simulink model "swing_up_final"  (R2020b)
settings: Solver=FixedStepDiscrete  StartTime=0.0  StopTime=Inf  FixedStep=0.001  RelTol=1e-3  EnableMultiTasking=on
values from neighbouring files (symbols this model uses):
  alfaBest = sin(2*pi*tacc/Tperiod)    [demo.m]    (also in pendulo_modelo.m)
  Gtd = c2d(Gt,T,'Tustin')    [demo.m]    (also in pendulo_modelo.m)
  Robs = [1 0 ... (first row only)    [demo.m]    (also in pendulo_modelo.m)
  Xmax = 0.02    [demo.m]    (also in pendulo_modelo.m = 0.045)
  Xmin = -0.02    [demo.m]    (also in pendulo_modelo.m = -0.045)
undefined symbols (not defined in the file or in its folder): DiscIntNeverNeededParam, Discrete, Kservo2, Time
libraries: simulink x5, arduinolib x2, ctrlSharedLib x1
settings Model: SILPILModeSetting=veronly  ExtModeTrigDuration=2  Creator=aleca  LastModifiedBy=aleca
settings OptimizationCC: EnhancedBackFolding=on  PassReuseOutputArgsAs=Individual arguments  ZeroExternalMemoryAtStartup=off  ZeroInternalMemoryAtStartup=off  MaxStackSize=64  OptimizeBlockOrder=speed  DifferentSizesBufferReuse=on  OptimizationCustomize=off  EfficientTunableParamExpr=on
settings DebuggingCC: ParameterTunabilityLossMsg=error
settings HardwareCC: ProdBitPerInt=16  ProdBitPerPointer=16  ProdBitPerSizeT=16  ProdBitPerPtrDiffT=16  ProdLargestAtomicFloat=None  ProdWordSize=8  ProdHWDeviceType=Atmel->AVR  UseEmbeddedCoderFeatures=off  UseSimulinkCoderFeatures=off
settings SFSimCC: MATLABDynamicMemAlloc=off
settings RTWCC: Description=Embedded Coder  SystemTargetFile=ert.tlc  HardwareBoard=Arduino Mega 2560  TemplateMakefile=ert_default_tmf  Toolchain=Arduino AVR  BuildConfiguration=Faster Runs
settings CodeAppCC: ForceParamTrailComments=on  IgnoreCustomStorageClasses=off  OperatorAnnotations=on  SimulinkDataObjDesc=on  SFDataObjDesc=on  InsertBlockDesc=on
settings ERTTargetCC: SupportContinuousTime=on  SupportNonInlinedSFcns=on  SupportVariableSizeSignals=on  ExtModeStaticAllocSize=2048

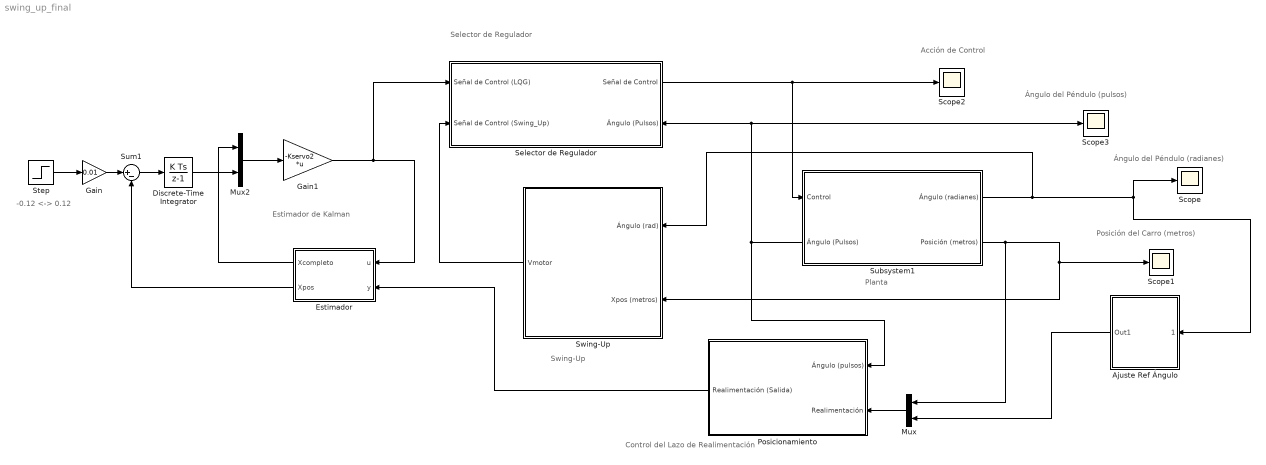
== system swing_up_final ==
  note: Selector de Regulador
  note: Posición del Carro (metros)
  note: Ángulo del Péndulo (radianes)
  note: Acción de Control
  note: Planta
  note: Ángulo del Péndulo (pulsos)
  note: Estimador de
      | Kalman
  note: Control del Lazo
      | de Realimentación
  note: -0.12 <-> 0.12
  note: Swing-Up
  Ajuste Ref Ángulo : Subsystem
  Discrete-Time Integrator : DiscreteIntegrator  SampleTime=-1  ICPrevOutput=DiscIntNeverNeededParam  ICPrevScaledInput=DiscIntNeverNeededParam
  Estimador : Subsystem
  Gain : Gain  Gain=0.01
  Gain1 : Gain  Gain=-Kservo2  Multiplication=Matrix(K*u)
  Mux : Mux  Inputs=2
  Mux2 : Mux  Inputs=2
  Posicionamiento : Subsystem
  Scope{,1..3} (4 alike) : Scope
  Selector de Regulador : Subsystem
      settings: PortSchema="{\"entries\":[{\"content\":{\"sides\":[{\"content\":{\"connectorIds\":[\"In1\",\"In2\"]},\"type\":\"ConnectorPlacement.EquallySpacedRectSide\",\"uuid\":\"3db4eb14-0c6e-4ec4-aee9-eaca3967a293\"},{\"content\":{\"connectorIds\":[\"Out1\",\"In3\"],\"side\":\"RIGHT\"},\"type\":\"ConnectorPlacement.EquallySpacedRectSide\",\"uuid\":\"3f8b5f83-bad3-4980-a559-890a6b6b79dc\"},{\"content\":{\"connectorIds\":[],\"side\":\"TOP\"},\"type\":\"ConnectorPlacement.EquallySpacedRectSide\",\"uuid\":\"0b873bda-4a27-449b-90e9-0421a7079439\"},{\"content\":{\"connectorIds\":[],\"side\":\"HIDDEN\"},\"type\":\"ConnectorPlacement.EquallySpacedRectSide\",\"uuid\":\"6335c064-abb3-4cb7-b774-07e736eb33ab\"}]},\"type\":\"ConnectorPlacement.EquallySpacedConnector\",\"uuid\":\"66807109-8b2f-4e1e-ad0b-5b86e298b8b1\"}],\"packageUris\":[\"http://schema.mathworks.com/mf0/Connector/R2020b\"],\"version\":\"1.0\"}"
  Step : Step  After=0  SampleTime=0.001
  Subsystem1 : Subsystem
      settings: PortSchema="{\"entries\":[{\"content\":{\"sides\":[{\"content\":{\"connectorIds\":[\"In1\",\"Out3\"]},\"type\":\"ConnectorPlacement.EquallySpacedRectSide\",\"uuid\":\"7b7d0a7e-b440-45e8-a961-32fe078fe659\"},{\"content\":{\"connectorIds\":[\"Out1\",\"Out2\"],\"side\":\"RIGHT\"},\"type\":\"ConnectorPlacement.EquallySpacedRectSide\",\"uuid\":\"86b71336-2b65-464f-a731-f6d3e5fd47fb\"},{\"content\":{\"connectorIds\":[],\"side\":\"TOP\"},\"type\":\"ConnectorPlacement.EquallySpacedRectSide\",\"uuid\":\"9d97f193-f97d-41ca-a241-68d679627dc2\"},{\"content\":{\"connectorIds\":[],\"side\":\"HIDDEN\"},\"type\":\"ConnectorPlacement.EquallySpacedRectSide\",\"uuid\":\"10f5410f-7265-49a9-9109-a49fd87294e3\"}]},\"type\":\"ConnectorPlacement.EquallySpacedConnector\",\"uuid\":\"71c4b2f0-2d03-4cb3-b067-cb634b3b5bca\"}],\"packageUris\":[\"http://schema.mathworks.com/mf0/Connector/R2020b\"],\"version\":\"1.0\"}"
  Sum1 : Sum  Inputs=|+-
  Swing-Up : Subsystem
      settings: PortSchema="{\"entries\":[{\"content\":{\"sides\":[{\"content\":{\"connectorIds\":[\"Out1\"]},\"type\":\"ConnectorPlacement.EquallySpacedRectSide\",\"uuid\":\"b2f1a7f6-c998-4070-93e8-aa818857c465\"},{\"content\":{\"connectorIds\":[\"In1\",\"In2\"],\"side\":\"RIGHT\"},\"type\":\"ConnectorPlacement.EquallySpacedRectSide\",\"uuid\":\"de419d1e-48dc-4c26-9042-5a784be48a2d\"},{\"content\":{\"connectorIds\":[],\"side\":\"TOP\"},\"type\":\"ConnectorPlacement.EquallySpacedRectSide\",\"uuid\":\"dc3aa332-44e8-4ab8-94b2-713354263e28\"},{\"content\":{\"connectorIds\":[],\"side\":\"HIDDEN\"},\"type\":\"ConnectorPlacement.EquallySpacedRectSide\",\"uuid\":\"62b3370c-add9-4815-8211-1f2eee1007cc\"}]},\"type\":\"ConnectorPlacement.EquallySpacedConnector\",\"uuid\":\"e08c5ebc-1d1c-48bb-8a56-91400baa4e78\"}],\"packageUris\":[\"http://schema.mathworks.com/mf0/Connector/R2020b\"],\"version\":\"1.0\"}"
  wires:
  Gain1/1 -> Selector de Regulador/1(Señal de Control (LQG)), Estimador/1(u)
  Selector de Regulador/1(Señal de Control) -> Subsystem1/1(Control), Scope2/1
  Estimador/2(Xpos) -> Sum1/2
  Mux/1 -> Posicionamiento/2(Realimentación)
  Estimador/1(Xcompleto) -> Mux2/1
  Gain/1 -> Sum1/1
  Subsystem1/3(Ángulo (Pulsos)) -> Scope3/1, Selector de Regulador/3(Ángulo (Pulsos)), Posicionamiento/1(Ángulo (pulsos))
  Mux2/1 -> Gain1/1
  Discrete-Time Integrator/1 -> Mux2/2
  Step/1 -> Gain/1
  Subsystem1/1(Ángulo (radianes)) -> Ajuste Ref Ángulo/1(1), Scope/1, Swing-Up/1(Ángulo (rad))
  Sum1/1 -> Discrete-Time Integrator/1
  Ajuste Ref Ángulo/1(Out1) -> Mux/2
  Posicionamiento/1(Realimentación (Salida)) -> Estimador/2(y)
  Subsystem1/2(Posición (metros)) -> Mux/1, Swing-Up/2(Xpos (metros)), Scope1/1
  Swing-Up/1(Vmotor) -> Selector de Regulador/2(Señal de Control (Swing_Up))

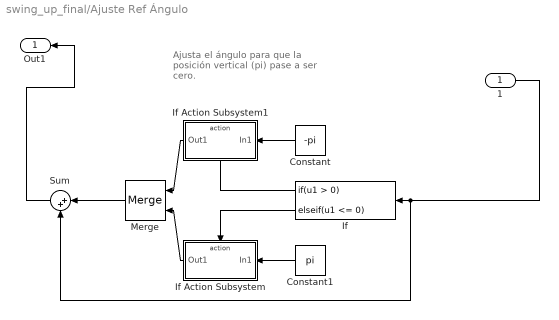
== system swing_up_final/Ajuste Ref Ángulo ==
  note: Ajusta el ángulo para que la posición vertical (pi) pase a ser cero.
  1 : Inport
  Constant : Constant  Value=-pi  SampleTime=0.001
  Constant1 : Constant  Value=pi  SampleTime=0.001
  If : If  ElseIfExpressions=u1 <= 0  ShowElse=off
  If Action Subsystem : Subsystem  TreatAsAtomicUnit=on
  If Action Subsystem1 : Subsystem  TreatAsAtomicUnit=on
  Merge : Merge
  Sum : Sum  Inputs=|++
  Out1 : Outport
  wires:
  Sum/1 -> Out1/1
  If Action Subsystem/1(Out1) -> Merge/2
  Constant/1 -> If Action Subsystem1/1(In1)
  If Action Subsystem1/1(Out1) -> Merge/1
  If/2 -> If Action Subsystem/Action
  Merge/1 -> Sum/1
  Constant1/1 -> If Action Subsystem/1(In1)
  If/1 -> If Action Subsystem1/Action
  1/1 -> Sum/2, If/1

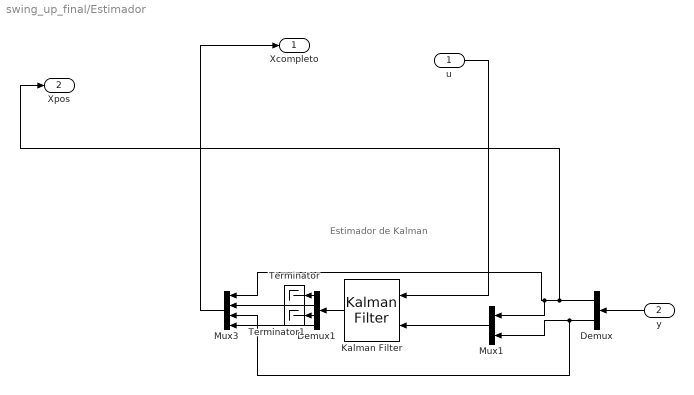
== system swing_up_final/Estimador ==
  note: Estimador
      | de Kalman
  u : Inport
  y : Inport  Port=2
  Demux : Demux  Outputs=2
  Demux1 : Demux
  Kalman Filter : ctrlSharedLib/Kalman Filter  TimeDomain=Discrete-Time  UseCurrentEstimator=off  ModelSource=Individual A, B, C, D matrices  ModelSourceVariable=ss(0.95,1,1,0,1)  A=Gtd.A  B=Gtd.B  C=Gtd.C  D=Gtd.D  NumberOfStates=1  NumberOfInputs=1  NumberOfOutputs=1  InitialEstimateSource=Dialog  X0=0  P0=10  UseK=off  UseGH=off  NumberOfProcessNoiseInputs=1  G=1  TimeInvariantG=on  H=0  TimeInvariantH=on  Q=Qobs  TimeInvariantQ=on  R=Robs  TimeInvariantR=on  N=0  TimeInvariantN=on  AddInputPort=on  AddEnablePort=off  OutputEstimatedY=off  OutputP=off  Ts=-1
  Mux1 : Mux  Inputs=2
  Mux3 : Mux
  Terminator : Terminator
  Terminator1 : Terminator
  Xcompleto : Outport
  Xpos : Outport  Port=2
  wires:
  Mux3/1 -> Xcompleto/1
  y/1 -> Demux/1
  Demux/1 -> Mux3/1, Mux1/1, Xpos/1
  Demux1/1 -> Terminator/1
  u/1 -> Kalman Filter/1
  Demux1/4 -> Mux3/4
  Kalman Filter/1 -> Demux1/1
  Demux1/2 -> Mux3/2
  Demux1/3 -> Terminator1/1
  Mux1/1 -> Kalman Filter/2
  Demux/2 -> Mux3/3, Mux1/2

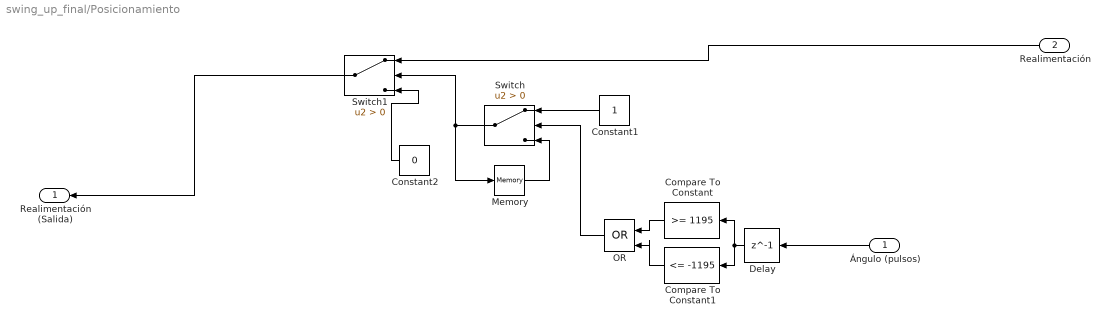
== system swing_up_final/Posicionamiento ==
  Ángulo (pulsos) : Inport
  Realimentación : Inport  Port=2
  Compare To Constant : simulink/Logic and Bit Operations/Compare To Constant  relop=>=  const=1195  OutDataTypeStr=boolean
  Compare To Constant1 : simulink/Logic and Bit Operations/Compare To Constant  relop=<=  const=-1195  OutDataTypeStr=boolean
  Constant1 : Constant  OutDataTypeStr=boolean  SampleTime=-1
  Constant2 : Constant  Value=0  SampleTime=-1
  Delay : Delay  DelayLength=1
  Memory : Memory  InheritSampleTime=on
  OR : Logic  Operator=OR  IconShape=distinctive  AllPortsSameDT=off  OutDataTypeStr=boolean
  Switch : Switch  Criteria=u2 > Threshold
  Switch1 : Switch  Criteria=u2 > Threshold
  Realimentación (Salida) : Outport
  wires:
  Memory/1 -> Switch/3
  Switch/1 -> Switch1/2, Memory/1
  Compare To Constant1/1 -> OR/2
  Compare To Constant/1 -> OR/1
  Delay/1 -> Compare To Constant/1, Compare To Constant1/1
  Constant2/1 -> Switch1/3
  OR/1 -> Switch/2
  Constant1/1 -> Switch/1
  Switch1/1 -> Realimentación (Salida)/1
  Ángulo (pulsos)/1 -> Delay/1
  Realimentación/1 -> Switch1/1

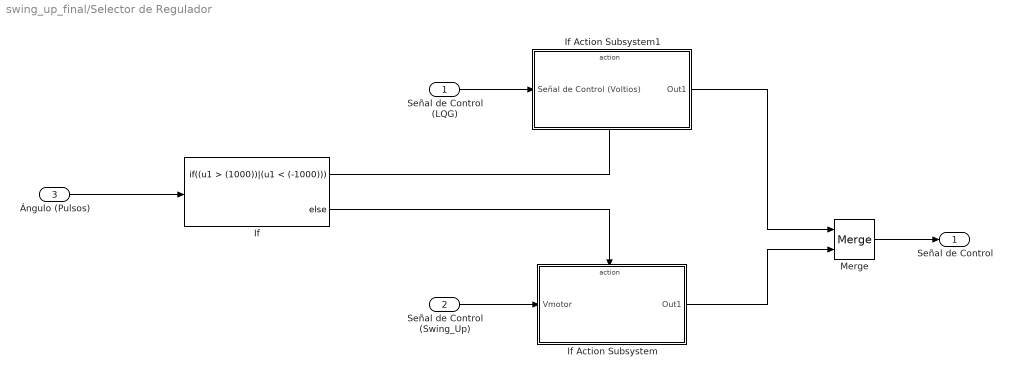
== system swing_up_final/Selector de Regulador ==
  Señal de Control (LQG) : Inport
  Señal de Control (Swing_Up) : Inport  Port=2
  Ángulo (Pulsos) : Inport  Port=3
  If : If  IfExpression=(u1 > (1000))|(u1 < (-1000))
  If Action Subsystem : Subsystem  TreatAsAtomicUnit=on
  If Action Subsystem1 : Subsystem  TreatAsAtomicUnit=on
  Merge : Merge
  Señal de Control : Outport
  wires:
  If Action Subsystem1/1(Out1) -> Merge/1
  Señal de Control (LQG)/1 -> If Action Subsystem1/1(Señal de Control (Voltios))
  If Action Subsystem/1(Out1) -> Merge/2
  Señal de Control (Swing_Up)/1 -> If Action Subsystem/1(Vmotor)
  Merge/1 -> Señal de Control/1
  If/1 -> If Action Subsystem1/Action
  If/2 -> If Action Subsystem/Action
  Ángulo (Pulsos)/1 -> If/1

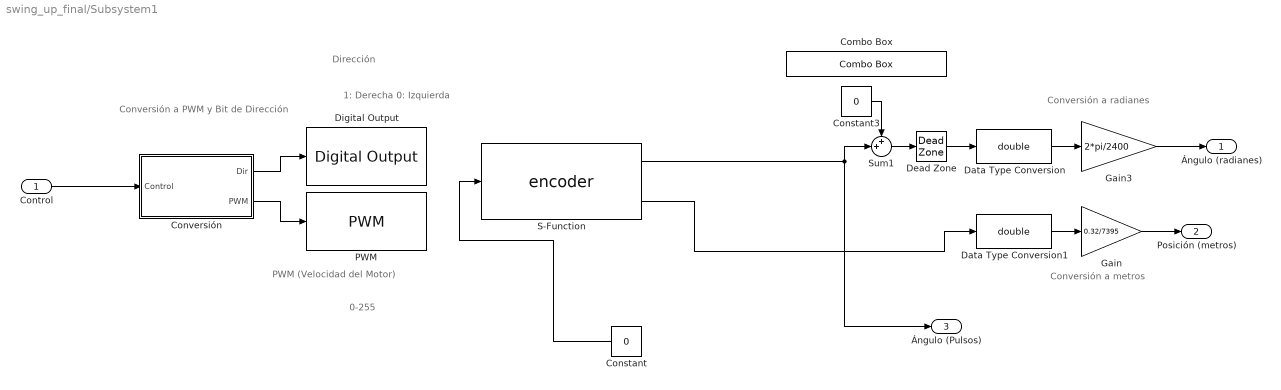
== system swing_up_final/Subsystem1 ==
  note: Conversión a metros
  note: Dirección
  note: PWM (Velocidad del Motor)
  note: 1: Derecha
      | 0: Izquierda
  note: Conversión a radianes
  note: 0-255
  note: Conversión a PWM y
      | Bit de Dirección
  Control : Inport
  Combo Box : ComboBox  LabelPosition=Hide  SelectedLabel=0
      settings: Values={{'0', '1', '2', '-2', '-1'}, [0 1 2 -2 -1]}
  Constant : Constant  Value=0  OutDataTypeStr=boolean  SampleTime=0.001
  Constant3 : Constant  Value=0  SampleTime=0.001
  Conversión : Subsystem
  Data Type Conversion : DataTypeConversion  OutDataTypeStr=double
  Data Type Conversion1 : DataTypeConversion  OutDataTypeStr=double
  Dead Zone : DeadZone  LowerValue=0  UpperValue=0  SaturateOnIntegerOverflow=on
  Digital Output : arduinolib/Digital Output  pinNumber=10  Direction=output  blockPlatform=arduino
  Gain : Gain  Gain=0.32/7395
  Gain3 : Gain  Gain=2*pi/2400
  PWM : arduinolib/PWM  pinNumber=9  frequencyType=Default  desiredFrequency=490.2  achievableFrequency=490.2
  S-Function : S-Function  FunctionName=encoder  SFunctionModules='encoder_wrapper'  SFunctionDeploymentMode=off  EnableBusSupport=off
  Sum1 : Sum  Inputs=++|
  Ángulo (radianes) : Outport
  Posición (metros) : Outport  Port=2
  Ángulo (Pulsos) : Outport  Port=3
  wires:
  Gain/1 -> Posición (metros)/1
  Sum1/1 -> Dead Zone/1
  Conversión/1(Dir) -> Digital Output/1
  Conversión/2(PWM) -> PWM/1
  Dead Zone/1 -> Data Type Conversion/1
  Data Type Conversion/1 -> Gain3/1
  Constant3/1 -> Sum1/1
  S-Function/2 -> Data Type Conversion1/1
  Data Type Conversion1/1 -> Gain/1
  Constant/1 -> S-Function/1
  Control/1 -> Conversión/1(Control)
  Gain3/1 -> Ángulo (radianes)/1
  S-Function/1 -> Ángulo (Pulsos)/1, Sum1/2

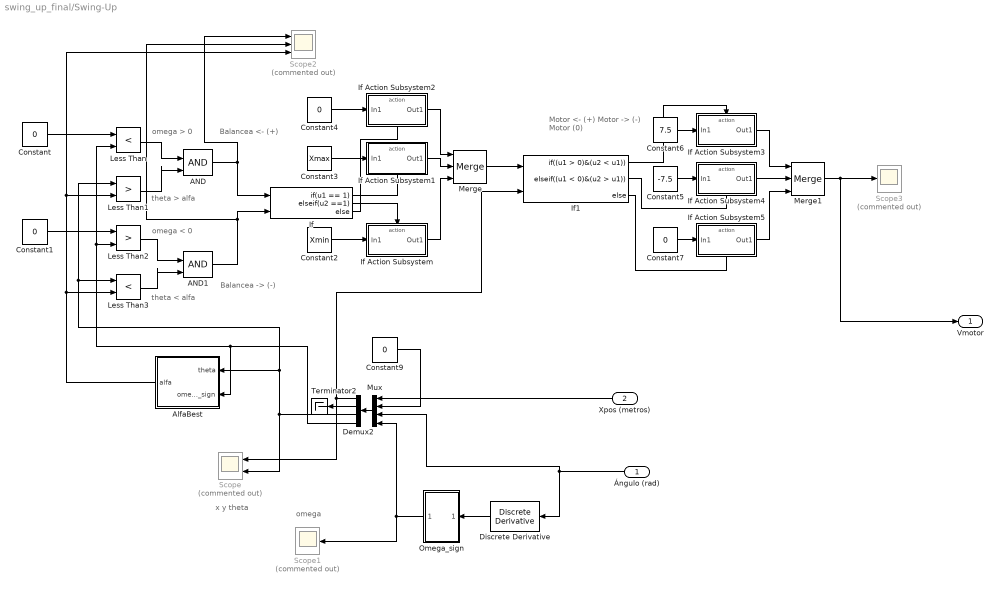
== system swing_up_final/Swing-Up ==
  note: x y theta
  note: omega
  note: Motor <- (+)
      | Motor -> (-)
      | Motor (0)
  note: Balancea -> (-)
  note: theta > alfa
  note: omega > 0
  note: omega < 0
  note: theta < alfa
  note: Balancea <- (+)
  Ángulo (rad) : Inport
  Xpos (metros) : Inport  Port=2
  AND : Logic  IconShape=distinctive  AllPortsSameDT=off  OutDataTypeStr=boolean
  AND1 : Logic  IconShape=distinctive  AllPortsSameDT=off  OutDataTypeStr=boolean
  AlfaBest : Subsystem
      settings: PortSchema="{\"entries\":[{\"content\":{\"sides\":[{\"content\":{\"connectorIds\":[\"Out1\"]},\"type\":\"ConnectorPlacement.EquallySpacedRectSide\",\"uuid\":\"f269d330-2dbf-4a03-aae2-9d91e46d5f46\"},{\"content\":{\"connectorIds\":[\"In1\",\"In2\"],\"side\":\"RIGHT\"},\"type\":\"ConnectorPlacement.EquallySpacedRectSide\",\"uuid\":\"83605d16-f426-4f00-b326-dfdad5d6c839\"},{\"content\":{\"connectorIds\":[],\"side\":\"TOP\"},\"type\":\"ConnectorPlacement.EquallySpacedRectSide\",\"uuid\":\"8003ed59-a4ef-474d-85bb-f26d1ffabd7e\"},{\"content\":{\"connectorIds\":[],\"side\":\"HIDDEN\"},\"type\":\"ConnectorPlacement.EquallySpacedRectSide\",\"uuid\":\"ae6ea9e2-c2fb-4e9e-9ec9-1e561a8d4724\"}]},\"type\":\"ConnectorPlacement.EquallySpacedConnector\",\"uuid\":\"f5174008-485c-4d77-9a7a-ef1ea74262ea\"}],\"packageUris\":[\"http://schema.mathworks.com/mf0/Connector/R2020b\"],\"version\":\"1.0\"}"
  Constant{,1,4,7,9} (5 alike) : Constant  Value=0  SampleTime=0.001
  Constant2 : Constant  Value=Xmin  SampleTime=0.001
  Constant3 : Constant  Value=Xmax  SampleTime=0.001
  Constant5 : Constant  Value=-7.5  SampleTime=0.001
  Constant6 : Constant  Value=7.5  SampleTime=0.001
  Demux2 : Demux
  Discrete Derivative : simulink/Discrete/Discrete Derivative  gainval=1.0  ICPrevScaledInput=0.0  OutMin=[]  OutMax=[]  OutDataType=fixdt(1, 16)  OutScaling=2^-10  DoSatur=off
  If : If  NumInputs=2  IfExpression=u1 == 1  ElseIfExpressions=u2 ==1
  If Action Subsystem : Subsystem  TreatAsAtomicUnit=on
  If Action Subsystem1 : Subsystem  TreatAsAtomicUnit=on
  If Action Subsystem2 : Subsystem  TreatAsAtomicUnit=on
  If Action Subsystem3 : Subsystem  TreatAsAtomicUnit=on
  If Action Subsystem4 : Subsystem  TreatAsAtomicUnit=on
  If Action Subsystem5 : Subsystem  TreatAsAtomicUnit=on
  If1 : If  NumInputs=2  IfExpression=(u1 > 0)&(u2 < u1)  ElseIfExpressions=(u1 < 0)&(u2 > u1)
  Less Than : RelationalOperator  Operator=<  OutDataTypeStr=boolean  RndMeth=Simplest
  Less Than1 : RelationalOperator  Operator=>  OutDataTypeStr=boolean  RndMeth=Simplest
  Less Than2 : RelationalOperator  Operator=>  OutDataTypeStr=boolean  RndMeth=Simplest
  Less Than3 : RelationalOperator  Operator=<  OutDataTypeStr=boolean  RndMeth=Simplest
  Merge : Merge  Inputs=3
  Merge1 : Merge  Inputs=3
  Mux : Mux
  Omega_sign : Subsystem
  Scope : Scope  Commented=on  NumInputPorts=2
  Scope1 : Scope  Commented=on
  Scope2 : Scope  Commented=on  NumInputPorts=3
  Scope3 : Scope  Commented=on
  Terminator2 : Terminator
  Vmotor : Outport
  wires:
  Constant3/1 -> If Action Subsystem1/1(In1)
  Less Than1/1 -> AND/2
  AND1/1 -> If/2, Scope2/2
  Omega_sign/1(Out1) -> Scope1/1, Mux/4
  Less Than/1 -> AND/1
  If Action Subsystem5/1(Out1) -> Merge1/3
  Constant1/1 -> Less Than2/1
  Less Than2/1 -> AND1/1
  Constant/1 -> Less Than/1
  If Action Subsystem3/1(Out1) -> Merge1/1
  AND/1 -> Scope2/1, If/1
  Demux2/3 -> Scope/2, Less Than3/1, Less Than1/1, AlfaBest/1(theta)
  Mux/1 -> Demux2/1
  If1/1 -> If Action Subsystem3/Action
  If Action Subsystem2/1(Out1) -> Merge/1
  Constant4/1 -> If Action Subsystem2/1(In1)
  Less Than3/1 -> AND1/2
  AlfaBest/1(alfa) -> Scope2/3, Less Than1/2, Less Than3/2
  Constant5/1 -> If Action Subsystem4/1(In1)
  Constant9/1 -> Mux/2
  Demux2/2 -> Terminator2/1
  Ángulo (rad)/1 -> Mux/3, Discrete Derivative/1
  Demux2/4 -> AlfaBest/2(omega_sign), Less Than/2, Less Than2/2
  Demux2/1 -> Scope/1, If1/2
  Constant7/1 -> If Action Subsystem5/1(In1)
  If/2 -> If Action Subsystem/Action
  Constant2/1 -> If Action Subsystem/1(In1)
  Merge1/1 -> Vmotor/1, Scope3/1
  Constant6/1 -> If Action Subsystem3/1(In1)
  If1/3 -> If Action Subsystem5/Action
  If Action Subsystem/1(Out1) -> Merge/3
  If Action Subsystem4/1(Out1) -> Merge1/2
  Merge/1 -> If1/1
  Discrete Derivative/1 -> Omega_sign/1(In1)
  If/1 -> If Action Subsystem1/Action
  If/3 -> If Action Subsystem2/Action
  If Action Subsystem1/1(Out1) -> Merge/2
  If1/2 -> If Action Subsystem4/Action
  Xpos (metros)/1 -> Mux/1

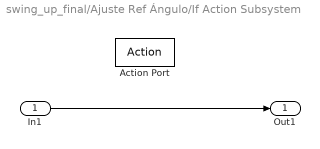
== system swing_up_final/Ajuste Ref Ángulo/If Action Subsystem ==
  In1 : Inport
  Action Port : ActionPort  ActionPortLabel=elseif(u1 <= 0)
  Out1 : Outport
  wires:
  In1/1 -> Out1/1

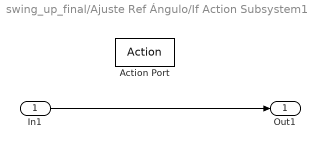
== system swing_up_final/Ajuste Ref Ángulo/If Action Subsystem1 ==
  In1 : Inport
  Action Port : ActionPort  ActionPortLabel=if(u1 > 0)
  Out1 : Outport
  wires:
  In1/1 -> Out1/1

== system swing_up_final/Selector de Regulador/If Action Subsystem ==
  Vmotor : Inport
  Action Port : ActionPort  ActionPortLabel=else
  Out1 : Outport
  wires:
  Vmotor/1 -> Out1/1

== system swing_up_final/Selector de Regulador/If Action Subsystem1 ==
  Señal de Control (Voltios) : Inport
  Action Port : ActionPort  ActionPortLabel=if((u1 > (1000))|(u1 < (-1000)))
  Out1 : Outport
  wires:
  Señal de Control (Voltios)/1 -> Out1/1

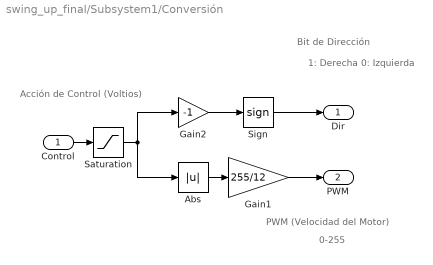
== system swing_up_final/Subsystem1/Conversión ==
  note: Acción de Control
      | (Voltios)
  note: Bit de Dirección
  note: 1: Derecha
      | 0: Izquierda
  note: 0-255
  note: PWM (Velocidad del Motor)
  Control : Inport
  Abs : Abs
  Gain1 : Gain  Gain=255/12
  Gain2 : Gain  Gain=-1
  Saturation : Saturate  UpperLimit=12  LowerLimit=-12
  Sign : Signum
  Dir : Outport
  PWM : Outport  Port=2
  wires:
  Abs/1 -> Gain1/1
  Gain1/1 -> PWM/1
  Control/1 -> Saturation/1
  Saturation/1 -> Gain2/1, Abs/1
  Sign/1 -> Dir/1
  Gain2/1 -> Sign/1

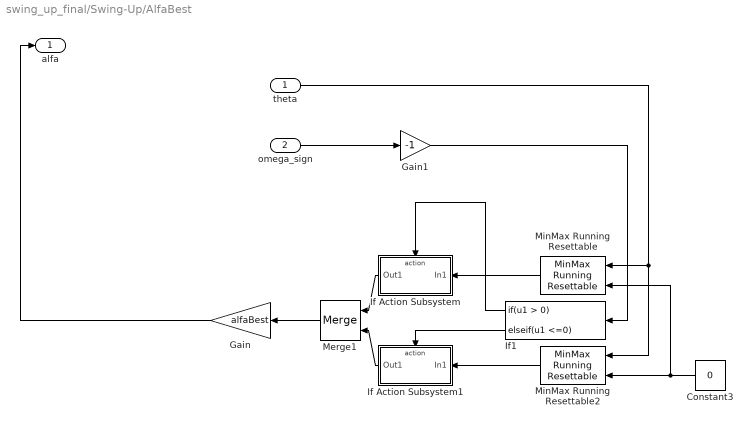
== system swing_up_final/Swing-Up/AlfaBest ==
  theta : Inport
  omega_sign : Inport  Port=2
  Constant3 : Constant  Value=0
  Gain : Gain  Gain=alfaBest
  Gain1 : Gain  Gain=-1
  If Action Subsystem : Subsystem  TreatAsAtomicUnit=on
  If Action Subsystem1 : Subsystem  TreatAsAtomicUnit=on
  If1 : If  ElseIfExpressions=u1 <=0  ShowElse=off
  Merge1 : Merge
  MinMax Running Resettable : simulink/Math Operations/MinMax Running Resettable  Function=max  vinit=0.0
  MinMax Running Resettable2 : simulink/Math Operations/MinMax Running Resettable  Function=min  vinit=0.0
  alfa : Outport
  wires:
  Constant3/1 -> MinMax Running Resettable/2, MinMax Running Resettable2/2
  If Action Subsystem1/1(Out1) -> Merge1/2
  theta/1 -> MinMax Running Resettable2/1, MinMax Running Resettable/1
  MinMax Running Resettable2/1 -> If Action Subsystem1/1(In1)
  If1/1 -> If Action Subsystem/Action
  Merge1/1 -> Gain/1
  Gain/1 -> alfa/1
  MinMax Running Resettable/1 -> If Action Subsystem/1(In1)
  If Action Subsystem/1(Out1) -> Merge1/1
  If1/2 -> If Action Subsystem1/Action
  omega_sign/1 -> Gain1/1
  Gain1/1 -> If1/1

== system swing_up_final/Swing-Up/If Action Subsystem ==
  In1 : Inport
  Action Port : ActionPort  ActionPortLabel=elseif(u2 ==1)
  Out1 : Outport
  wires:
  In1/1 -> Out1/1

== system swing_up_final/Swing-Up/If Action Subsystem1 ==
  In1 : Inport
  Action Port : ActionPort  ActionPortLabel=if(u1 == 1)
  Out1 : Outport
  wires:
  In1/1 -> Out1/1

== system swing_up_final/Swing-Up/If Action Subsystem2 ==
  In1 : Inport
  Action Port : ActionPort  ActionPortLabel=else
  Out1 : Outport
  wires:
  In1/1 -> Out1/1

== system swing_up_final/Swing-Up/If Action Subsystem3 ==
  In1 : Inport
  Action Port : ActionPort  ActionPortLabel=if((u1 > 0)&(u2 < u1))
  Out1 : Outport
  wires:
  In1/1 -> Out1/1

== system swing_up_final/Swing-Up/If Action Subsystem4 ==
  In1 : Inport
  Action Port : ActionPort  ActionPortLabel=elseif((u1 < 0)&(u2 > u1))
  Out1 : Outport
  wires:
  In1/1 -> Out1/1

== system swing_up_final/Swing-Up/If Action Subsystem5 ==
  In1 : Inport
  Action Port : ActionPort  ActionPortLabel=else
  Out1 : Outport
  wires:
  In1/1 -> Out1/1

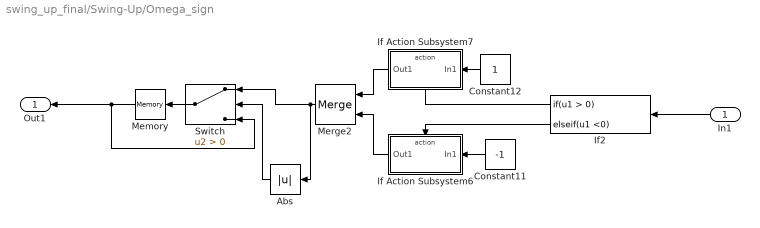
== system swing_up_final/Swing-Up/Omega_sign ==
  In1 : Inport
  Abs : Abs
  Constant11 : Constant  Value=-1  SampleTime=0.001
  Constant12 : Constant  SampleTime=0.001
  If Action Subsystem6 : Subsystem  TreatAsAtomicUnit=on
  If Action Subsystem7 : Subsystem  TreatAsAtomicUnit=on
  If2 : If  ElseIfExpressions=u1 <0  ShowElse=off
  Memory : Memory
  Merge2 : Merge
  Switch : Switch  Criteria=u2 > Threshold
  Out1 : Outport
  wires:
  In1/1 -> If2/1
  If Action Subsystem6/1(Out1) -> Merge2/2
  Merge2/1 -> Abs/1, Switch/1
  Abs/1 -> Switch/2
  If2/1 -> If Action Subsystem7/Action
  If Action Subsystem7/1(Out1) -> Merge2/1
  If2/2 -> If Action Subsystem6/Action
  Memory/1 -> Out1/1, Switch/3
  Switch/1 -> Memory/1
  Constant12/1 -> If Action Subsystem7/1(In1)
  Constant11/1 -> If Action Subsystem6/1(In1)

== system swing_up_final/Swing-Up/AlfaBest/If Action Subsystem ==
  In1 : Inport
  Action Port : ActionPort  ActionPortLabel=if(u1 > 0)
  Out1 : Outport
  wires:
  In1/1 -> Out1/1

== system swing_up_final/Swing-Up/AlfaBest/If Action Subsystem1 ==
  In1 : Inport
  Action Port : ActionPort  ActionPortLabel=elseif(u1 <=0)
  Out1 : Outport
  wires:
  In1/1 -> Out1/1

== system swing_up_final/Swing-Up/Omega_sign/If Action Subsystem6 ==
  In1 : Inport
  Action Port : ActionPort  ActionPortLabel=elseif(u1 <0)
  Out1 : Outport
  wires:
  In1/1 -> Out1/1

== system swing_up_final/Swing-Up/Omega_sign/If Action Subsystem7 ==
  In1 : Inport
  Action Port : ActionPort  ActionPortLabel=if(u1 > 0)
  Out1 : Outport
  wires:
  In1/1 -> Out1/1
